simulink model "FrequencyModulation"  (R2023b)
settings: Solver=VariableStepAuto  StartTime=0.0  StopTime=10.0  RelTol=1e-3
settings Model: Creator=satyamagrawal  LastModifiedBy=satyamagrawal

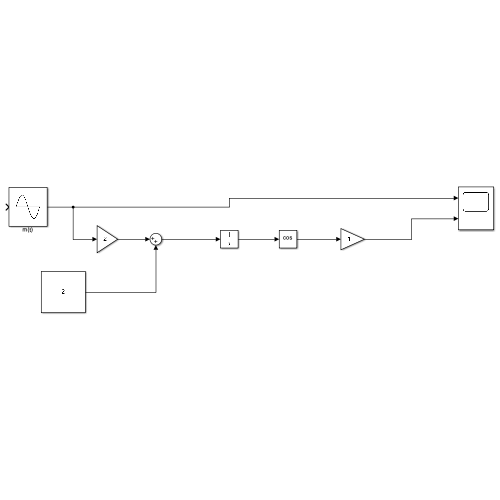
[thumbnail: Simulink's stored preview of the top-level diagram]
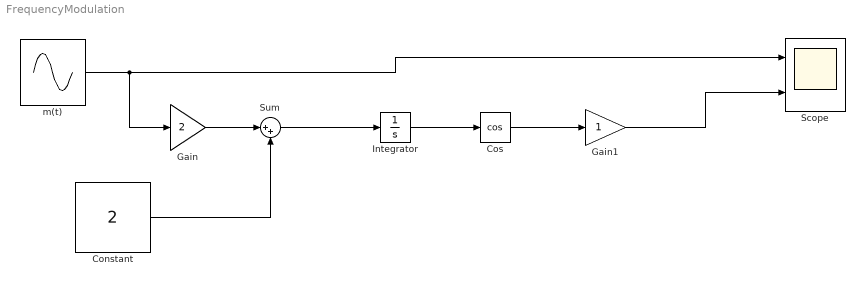
== system FrequencyModulation ==
  Constant : Constant  Value=2
  Cos : Trigonometry  Operator=cos
  Gain : Gain  Gain=2
  Gain1 : Gain
  Integrator : Integrator
  Scope : Scope  NumInputPorts=2
  Sum : Sum  Inputs=|++
  m(t) : Sin  TimeSource=Use external signal  Frequency=10  SampleTime=0
  wires:
  m(t)/1 -> Gain/1, Scope/1
  Sum/1 -> Integrator/1
  Gain/1 -> Sum/1
  Gain1/1 -> Scope/2
  Constant/1 -> Sum/2
  Integrator/1 -> Cos/1
  Cos/1 -> Gain1/1
